simulink model "BLOC_Power_efficiency"  (R2016a)
settings: Solver=FixedStepDiscrete  StartTime=0.0  StopTime=10.0  FixedStep=hev_dt  RelTol=1e-3
undefined symbols (not defined in the file): hev_dt, ra_electrical_machine_efficiency, ra_electrical_machine_speed, ra_electrical_machine_torque
settings Model: Creator=Florent  LastModifiedBy=Florent
settings OptimizationCC: DefaultParameterBehavior=Inlined  OptimizeModelRefInitCode=on  LifeSpan=1
settings RTWCC: SystemTargetFile=ert.tlc  TemplateMakefile=ert_default_tmf  GenerateReport=on  IncludeHyperlinkInReport=on  LaunchReport=on  TargetLang=C++  GenerateTraceInfo=on  GenerateTraceReport=on  GenerateTraceReportSl=on  GenerateTraceReportSf=on  GenerateTraceReportEml=on
settings CodeAppCC: ForceParamTrailComments=on  OperatorAnnotations=on  SimulinkDataObjDesc=on  SFDataObjDesc=on  MATLABFcnDesc=on  InsertBlockDesc=on  MATLABSourceComments=on
settings ERTTargetCC: GenerateSampleERTMain=on  MultiInstanceERTCode=on  CodeInterfacePackaging=C++ class  InlinedParameterPlacement=NonHierarchical  RootIOFormat=Structure reference  ERTCustomFileTemplate=example_file_process.tlc

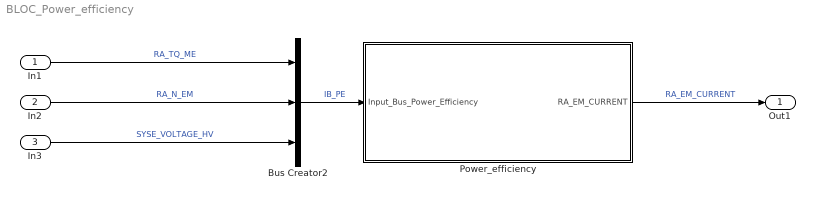
== system BLOC_Power_efficiency ==
  In1 : Inport
  In2 : Inport  Port=2
  In3 : Inport  Port=3
  Bus Creator2 : BusCreator  Inputs=3
  Power_efficiency : Subsystem  TreatAsAtomicUnit=on  SystemSampleTime=hev_dt
  Out1 : Outport
  wires:
  Power_efficiency/1(RA_EM_CURRENT) -> Out1/1  "RA_EM_CURRENT"
  Bus Creator2/1 -> Power_efficiency/1(Input_Bus_Power_Efficiency)  "IB_PE"
  In1/1 -> Bus Creator2/1  "RA_TQ_ME"
  In2/1 -> Bus Creator2/2  "RA_N_EM"
  In3/1 -> Bus Creator2/3  "SYSE_VOLTAGE_HV"

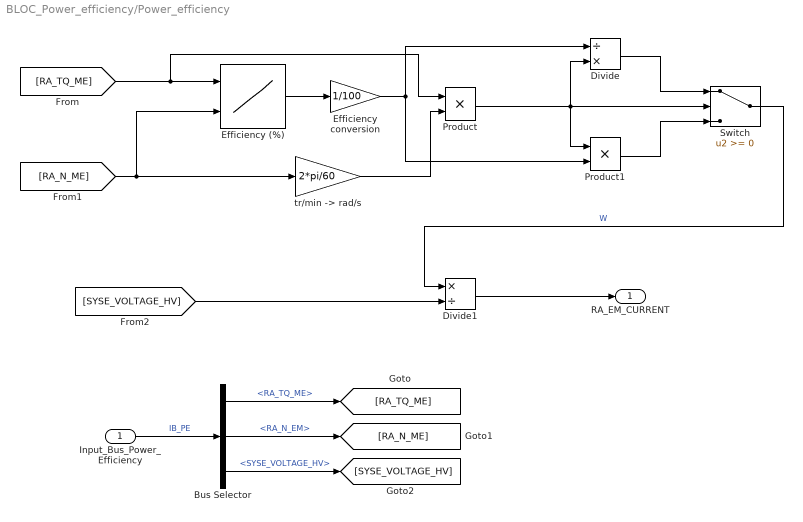
== system BLOC_Power_efficiency/Power_efficiency ==
  Input_Bus_Power_Efficiency : Inport
  Bus Selector : BusSelector  OutputSignals=RA_TQ_ME,RA_N_EM,SYSE_VOLTAGE_HV
  Divide : Product  Inputs=/*  SampleTime=hev_dt
  Divide1 : Product  Inputs=*/  SampleTime=hev_dt
  Efficiency (%) : Lookup_n-D  BreakpointsForDimension1=ra_electrical_machine_torque  BreakpointsForDimension2=ra_electrical_machine_speed  Table=ra_electrical_machine_efficiency  SampleTime=hev_dt  RndMeth=Simplest  InputSameDT=on
  Efficiency conversion : Gain  Gain=1/100  SampleTime=hev_dt
  Product : Product  SampleTime=hev_dt  RndMeth=Zero
  Product1 : Product  SampleTime=hev_dt  RndMeth=Zero
  Switch : Switch  SampleTime=hev_dt
  "tr/min -> rad/s" : Gain  Gain=2*pi/60  SampleTime=hev_dt
  RA_EM_CURRENT : Outport
  wires:
  Efficiency (%)/1 -> Efficiency conversion/1
  Product/1 -> Switch/2, Product1/1, Divide/2
  Divide/1 -> Switch/1
  Product1/1 -> Switch/3
  Efficiency conversion/1 -> Product1/2, Divide/1
  "tr/min -> rad/s"/1 -> Product/2
  Switch/1 -> Divide1/1  "W"
  [RA_TQ_ME] -> Product/1, Efficiency (%)/1
  [RA_N_ME] -> Efficiency (%)/2, "tr/min -> rad/s"/1
  Divide1/1 -> RA_EM_CURRENT/1
  [SYSE_VOLTAGE_HV] -> Divide1/2
  Input_Bus_Power_Efficiency/1 -> Bus Selector/1  "IB_PE"
  Bus Selector/1 -> [RA_TQ_ME]  "<RA_TQ_ME>"
  Bus Selector/2 -> [RA_N_ME]  "<RA_N_EM>"
  Bus Selector/3 -> [SYSE_VOLTAGE_HV]  "<SYSE_VOLTAGE_HV>"
